simulink model "CounterSF_Task"  (R2021a)
settings: Solver=FixedStepDiscrete  StartTime=0.0  StopTime=10.0  RelTol=1e-3
settings Model: Creator=Mohamed Elomda  LastModifiedBy=Mohamed Elomda
settings OptimizationCC: DefaultParameterBehavior=Inlined  EnhancedBackFolding=on  PassReuseOutputArgsAs=Individual arguments  ZeroExternalMemoryAtStartup=off  ZeroInternalMemoryAtStartup=off  OptimizeBlockOrder=speed  DifferentSizesBufferReuse=on  OptimizationCustomize=off  EfficientTunableParamExpr=on
settings DebuggingCC: UnderspecifiedInitializationDetection=Classic  MergeDetectMultiDrivingBlocksExec=none  ParameterTunabilityLossMsg=error
settings ModelReferenceCC: PropagateSignalLabelsOutOfModel=off
settings SFSimCC: MATLABDynamicMemAlloc=off
settings RTWCC: SystemTargetFile=ert.tlc  GenCodeOnly=on  TemplateMakefile=ert_default_tmf  GenerateReport=on  LaunchReport=on
settings CodeAppCC: ForceParamTrailComments=on  IgnoreCustomStorageClasses=off  OperatorAnnotations=on  SimulinkDataObjDesc=on  SFDataObjDesc=on  InsertBlockDesc=on
settings ERTTargetCC: TargetLangStandard=C99 (ISO)  GenerateSampleERTMain=on  InlinedParameterPlacement=NonHierarchical  ERTCustomFileTemplate=example_file_process.tlc

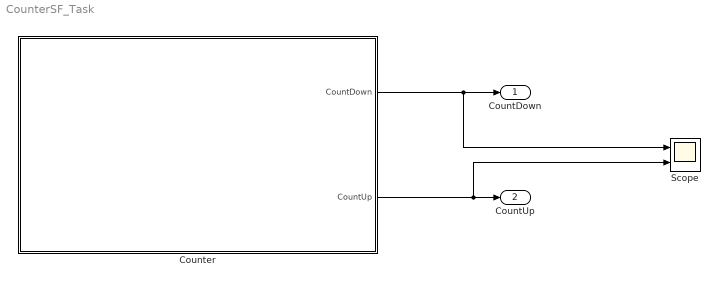
== system CounterSF_Task ==
  Counter : Stateflow chart  TreatAsAtomicUnit=on
      settings: RTWSystemCode=Reusable function  RTWFcnNameOpts=Use subsystem name  RTWFileNameOpts=Use subsystem name
  Scope : Scope  NumInputPorts=2
  CountDown : Outport
  CountUp : Outport  Port=2
  wires:
  Counter/2(CountUp) -> Scope/2, CountUp/1
  Counter/1(CountDown) -> Scope/1, CountDown/1

== stateflow chart CounterSF_Task/Counter ==
  state CountUp_And_Down_Modifier
    entry:
    CountUp = CountUp + 1;
    CountDown = CountDown - 1;
  state Reset
    entry:
    CountUp = 0;
    CountDown = 10;
  (default) -> CountUp_And_Down_Modifier
  CountUp_And_Down_Modifier -> CountUp_And_Down_Modifier [order 2] : after(1,tick)
  Reset -> CountUp_And_Down_Modifier
  CountUp_And_Down_Modifier -> Reset [order 1] : [CountUp == 10]
  data: CountDown output =11; CountUp output =-1
